simulink model "example_Hydraulic_PumpAdditional"  (R2018b)
settings: Solver=ode45  StartTime=0.0  StopTime=200  MaxStep=5  RelTol=1e-3  EnableMultiTasking=on
undefined symbols (not defined in the file): path_carnot
libraries: carnot x9, simulink x2
settings Model: Creator=drhf  LastModifiedBy=drhf
settings DataIOCC: LimitDataPoints=on  SaveFormat=Array  SignalLoggingSaveFormat=ModelDataLogs
settings OptimizationCC: ExpressionDepthLimit=2147483647  LifeSpan=inf
settings DebuggingCC: UnderspecifiedInitializationDetection=Classic  MergeDetectMultiDrivingBlocksExec=none  SolverPrmCheckMsg=warning  StateNameClashWarn=warning  SFUnexpectedBacktrackingDiag=warning  SFNoUnconditionalDefaultTransitionDiag=warning  SFExecutionAtInitializationDiag=none
settings HardwareCC: ProdBitPerPointer=32  ProdBitPerSizeT=32  ProdBitPerPtrDiffT=32  ProdLargestAtomicFloat=None  ProdIntDivRoundTo=Undefined  ProdEndianess=Unspecified  ProdWordSize=32  ProdHWDeviceType=32-bit Generic
settings ModelReferenceCC: PropagateSignalLabelsOutOfModel=off
settings SFSimCC: SimUseLocalCustomCode=off
settings RTWCC: RTWUseLocalCustomCode=off
settings CodeAppCC: StateflowObjectComments=on
settings GRTTargetCC: TargetLangStandard=C89/C90 (ANSI)  GeneratePreprocessorConditionals=Disable all  CombineOutputUpdateFcns=off  GRTInterface=on
settings ConfigComp: CovMetricSettings=dw  CovHtmlReporting=on  CovSaveCumulativeToWorkspaceVar=on  CovSaveSingleToWorkspaceVar=on  CovExternalEMLEnable=off

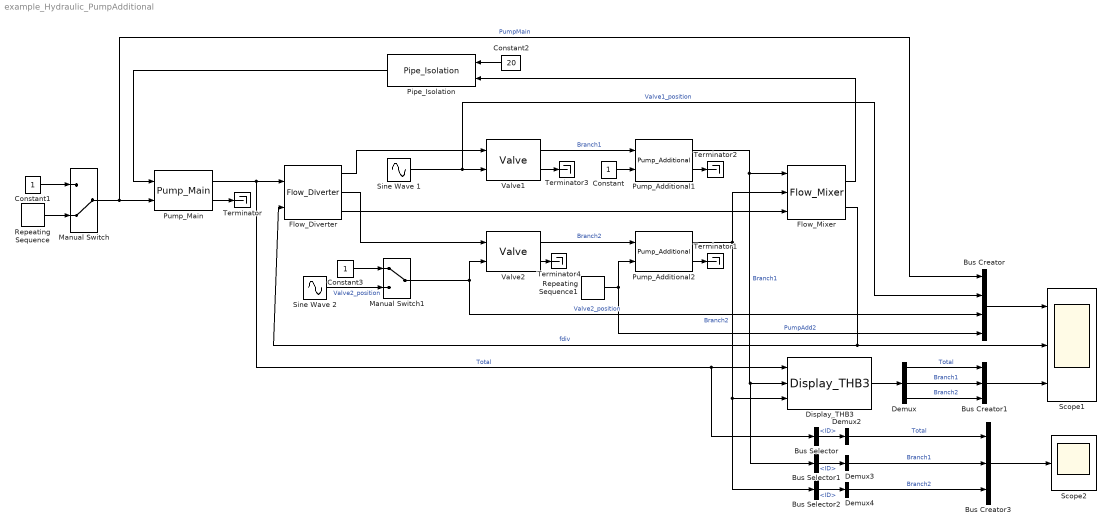
== system example_Hydraulic_PumpAdditional ==
  Bus Creator : BusCreator  Inputs=4
  Bus Creator1 : BusCreator  Inputs=3
  Bus Creator3 : BusCreator  Inputs=3
  Bus Selector : BusSelector  OutputSignals=ID
  Bus Selector1 : BusSelector  OutputSignals=ID
  Bus Selector2 : BusSelector  OutputSignals=ID
  Constant : Constant
  Constant1 : Constant
  Constant2 : Constant  Value=20
  Constant3 : Constant
  Demux : Demux  Outputs=3
  Demux2 : Demux  Outputs=1
  Demux3 : Demux  Outputs=1
  Demux4 : Demux  Outputs=1
  Display_THB3 : carnot/Outputs/Display_THB3  t=off  m=on  p=off  id=off  mix=off  d=off
      settings: SourceProductName=Carnot
  Flow_Diverter : carnot/Hydraulics/Flow_Diverter
      settings: SourceProductName=Carnot
  Flow_Mixer : carnot/Hydraulics/Flow_Mixer
      settings: SourceProductName=Carnot
  Manual Switch : ManualSwitch  CurrentSetting=0
  Manual Switch1 : ManualSwitch
  Pipe_Isolation : carnot/Hydraulics/Pipe_Isolation  dia=0.02  len=10  hgt=0  isolat=43.72  condiso=0.05  cond=0  cwall=1000  t0=20  lin=100/0.2  qua=100/0.2^2  nodes=10
      settings: SourceProductName=Carnot
  Pump_Additional1 : carnot/Hydraulics/Pump_Additional  Tini=20  PathName=fullfile(path_carnot('libsl'), 'Hydraulics', 'Pump_Main', 'parameter_set')  FileName='Pump5m.mat'  userPath=off  userParam=off  a0=50000  a1=-45000  a2=0  dia=0.025  UA=1  mcp=4182  e0=35  e1=22.5  e2=-8.1
      settings: SourceProductName=Carnot
  Pump_Additional2 : carnot/Hydraulics/Pump_Additional  Tini=20  PathName=fullfile(path_carnot('libsl'), 'Hydraulics', 'Pump_Main', 'parameter_set')  FileName='Pump4m.mat'  userPath=off  userParam=off  a0=40000  a1=-40000  a2=0  dia=0.02  UA=1  mcp=4182  e0=30  e1=25  e2=-10
      settings: SourceProductName=Carnot
  Pump_Main : carnot/Hydraulics/Pump_Main  Tini=20  p0=3e5  IDpreset=pressure drop  fluid=Water  mix=0  mix2=0  mix3=0  t1=0.1  PathName=fullfile(path_carnot('libsl'), 'Hydraulics', 'Pump_Main', 'parameter_set')  FileName='Pump5m.mat'  userPath=off  userParam=off  a0=50000  a1=-45000  a2=0  dia=0.025  UA=1  mcp=4182  e0=35  e1=22.5  e2=-8.1
      settings: SourceProductName=Carnot
  Repeating Sequence : simulink/Sources/Repeating Sequence  rep_seq_t=[0 20 60 200]  rep_seq_y=[0 0 1 1]
  Repeating Sequence1 : simulink/Sources/Repeating Sequence  rep_seq_t="[0 80 100  200]"  rep_seq_y=[0 0 1 1]
  Scope1 : Scope  NumInputPorts=3
  Scope2 : Scope
  Sine Wave 1 : Sin  Amplitude=0.6  Bias=0.5  Frequency=1/20  SampleTime=0
  Sine Wave 2 : Sin  Amplitude=0.6  Bias=0.5  Frequency=1/20  Phase=pi  SampleTime=0
  Terminator{,1..4} (5 alike) : Terminator
  Valve1 : carnot/Hydraulics/Valve  vtyp=linear  psi_0=0.04  kvs=1.6  dt_V=30
      settings: SourceProductName=Carnot
  Valve2 : carnot/Hydraulics/Valve  vtyp=linear  psi_0=0.04  kvs=1.6  dt_V=30
      settings: SourceProductName=Carnot
  wires:
  Pump_Additional2/2 -> Terminator1/1
  Pump_Additional1/2 -> Terminator2/1
  Manual Switch/1 -> Bus Creator/1, Pump_Main/2  "PumpMain"
  Pump_Main/2 -> Terminator/1
  Sine Wave 1/1 -> Valve1/2, Bus Creator/2  "Valve1_position"
  Flow_Diverter/1 -> Valve1/1
  Manual Switch1/1 -> Bus Creator/3, Valve2/2  "Valve2_position"
  Flow_Diverter/2 -> Valve2/1
  Flow_Diverter/3 -> Flow_Mixer/3
  Flow_Mixer/2 -> Flow_Diverter/2, Scope1/2  "fdiv"
  Flow_Mixer/1 -> Pipe_Isolation/2
  Bus Creator/1 -> Scope1/1
  Pump_Additional1/1 -> Bus Selector1/1, Display_THB3/2, Flow_Mixer/1  "Branch1"
  Pump_Additional2/1 -> Bus Selector2/1, Display_THB3/3, Flow_Mixer/2  "Branch2"
  Pump_Main/1 -> Flow_Diverter/1, Bus Selector/1, Display_THB3/1  "Total"
  Display_THB3/1 -> Demux/1
  Demux/1 -> Bus Creator1/1  "Total"
  Demux/2 -> Bus Creator1/2  "Branch1"
  Demux/3 -> Bus Creator1/3  "Branch2"
  Bus Creator1/1 -> Scope1/3
  Demux2/1 -> Bus Creator3/1  "Total"
  Demux4/1 -> Bus Creator3/3  "Branch2"
  Bus Creator3/1 -> Scope2/1
  Bus Selector/1 -> Demux2/1  "<ID>"
  Bus Selector1/1 -> Demux3/1  "<ID>"
  Demux3/1 -> Bus Creator3/2  "Branch1"
  Bus Selector2/1 -> Demux4/1  "<ID>"
  Valve1/1 -> Pump_Additional1/1  "Branch1"
  Constant/1 -> Pump_Additional1/2
  Valve2/1 -> Pump_Additional2/1  "Branch2"
  Repeating Sequence1/1 -> Bus Creator/4, Pump_Additional2/2  "PumpAdd2"
  Repeating Sequence/1 -> Manual Switch/2
  Constant1/1 -> Manual Switch/1
  Valve1/2 -> Terminator3/1
  Valve2/2 -> Terminator4/1
  Pipe_Isolation/1 -> Pump_Main/1
  Constant2/1 -> Pipe_Isolation/1
  Constant3/1 -> Manual Switch1/1
  Sine Wave 2/1 -> Manual Switch1/2  "Valve2_position"
